simulink model "ThreeDOF_Rocket_Simulator_v4_NEW"  (R2023b)
settings: Solver=VariableStepAuto  StartTime=0.0  StopTime=30  RelTol=1e-3
libraries: shared3dof x1, simulink_extras x1, simulink x1
settings Model: Creator=giuse  LastModifiedBy=matti
settings OptimizationCC: ReuseModelBlockBuffer=off
settings DebuggingCC: UnconnectedInputMsg=warning  UnconnectedOutputMsg=warning  UnconnectedLineMsg=warning
settings ModelReferenceCC: EnableRefExpFcnMdlSchedulingChecks=on
settings RTWCC: DLArmComputeVersion=19.05

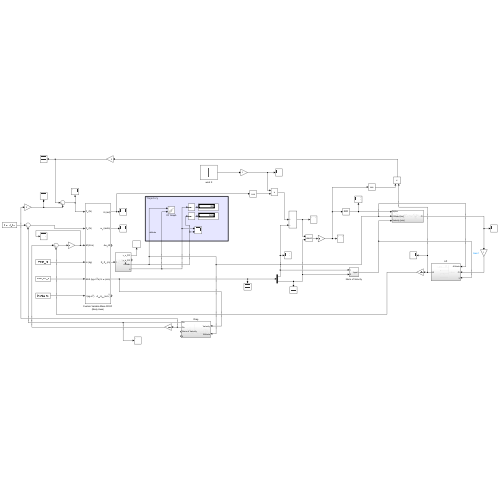
[thumbnail: Simulink's stored preview of the top-level diagram]
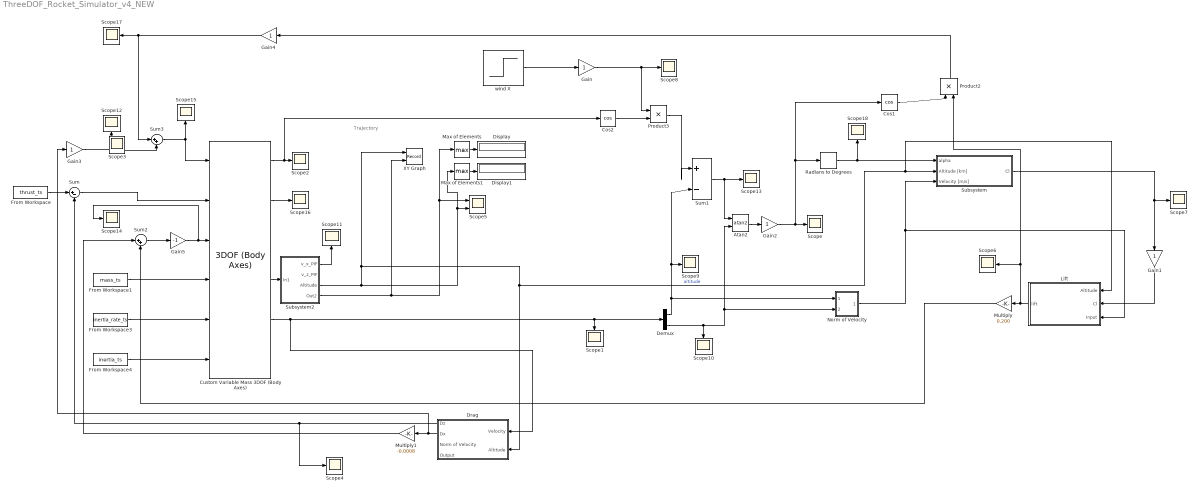
== system ThreeDOF_Rocket_Simulator_v4_NEW ==
  note: Trajectory
  Atan2 : Trigonometry  Operator=atan2
  Cos1 : Trigonometry  Operator=cos
  Cos2 : Trigonometry  Operator=cos
  Custom Variable Mass 3DOF (Body Axes) : shared3dof/3DOF (Body Axes)  units=Metric (MKS)  mtype=Custom Variable  v_ini=0  theta_ini=pi  alpha_ini=pi/2  pos_ini=[0 0]  q_ini=0  mass=1.0  mass_e=0.5  mass_f=3.0  Iyy=1.0  Iyy_e=0.5  Iyy_f=3.0  g_in=Internal  g=9.81  vre_flag=off  abi_flag=off  aMode=0  vel_statename=''  theta_statename=''  pos_statename=''  q_statename=''  mass_statename=''
  Demux : Demux  Outputs=2
  Display : Display
  Display1 : Display
  Drag : Subsystem
  From Workspace : FromWorkspace  VariableName=thrust_ts
  From Workspace1 : FromWorkspace  VariableName=mass_ts
  From Workspace3 : FromWorkspace  VariableName=inertia_rate_ts
  From Workspace4 : FromWorkspace  VariableName=inertia_ts
  Gain{,1..4} (5 alike) : Gain
  Gain5 : Gain  Gain=-1
  Lift : Subsystem
  Max of Elements : MinMax  Function=max
  Max of Elements1 : MinMax  Function=max
  Multiply : Gain  Gain=0.200
  Multiply1 : Gain  Gain=-0.0008
  Norm of Velocity : Subsystem
  Product2 : Product
  Product3 : Product
  Radians to Degrees : simulink_extras/Transformations/Radians to Degrees
  Scope{,1..4,6..18} (18 alike) : Scope
  Scope5 : Scope  NumInputPorts=2
  Subsystem : Subsystem
  Subsystem2 : Subsystem
  Sum : Sum  Inputs=|+-
  Sum1 : Sum  Inputs=|+-
  Sum2 : Sum  Inputs=|++
  Sum3 : Sum  Inputs=|++
  XY Graph : Record  FileSettingsInternal="{\"entries\":[{\"content\":{\"excelSettings\":{\"content\":{},\"type\":\"Streamout.ExcelSettings\"}},\"type\":\"Streamout.FileSettingStorage\",\"uuid\":\"\"}],\"packageUris\":[\"http:\\/\\/schema.mathworks.com\\/mf0\\/streamout_blocks\\/R2020a\"],\"version\":\"1.0\"}"  Layout=[1 1]  SignalsInternal="{\"entries\":[{\"content\":{\"signals\":[{\"content\":{\"blockPath\":[],\"dimensions\":[1],\"domain\":\"\",\"lineColor\":\"#0072bd\",\"plots\":[1],\"port\":1,\"sid\":[\"\"],\"signalID\":2529,\"signalName\":\"altitude\"},\"type\":\"RecordBlkView.Signal\",\"uuid\":\"\"},{\"content\":{\"blockPath\":[],\"dimensions\":[1],\"domain\":\"\",\"lineColor\":\"#d95319\",\"plots\":[1],\"port\":2,\"sid\":[\"\"],\"signalID\":2533,\"signalName\":\"Subsystem2:4\"},\"type\":\"RecordBlkView.Signal\",\"uuid\":\"\"}]},\"type\":\"RecordBlkView.InputSignals\",\"uuid\":\"\"}],\"packageUris\":[\"http:\\/\\/schema.mathworks.com\\/mf0\\/streamout_blocks\\/R2020a\"],\"version\":\"1.0\"}"  VisualizationBindings="{\"xyplotplugin\":{\"info\":[{\"series\":[{\"bindingParametersList\":[{\"parameter\":\"Y-Axis\",\"signalID\":2529,\"signalName\":\"altitude\"},{\"parameter\":\"X-Axis\",\"signalID\":2533,\"signalName\":\"Subsystem2:4\"}],\"seriesID\":11487}],\"subplotID\":1}]}}"  CompatibilityTag=XY
  wind X : Step  Time=0.357  After=-6  SampleTime=0
  wires:
  From Workspace1/1 -> Custom Variable Mass 3DOF (Body Axes)/4
  From Workspace4/1 -> Custom Variable Mass 3DOF (Body Axes)/6
  From Workspace/1 -> Sum/1
  Sum/1 -> Custom Variable Mass 3DOF (Body Axes)/2
  Sum2/1 -> Gain5/1
  Custom Variable Mass 3DOF (Body Axes)/4 -> Subsystem2/1(In1)
  Custom Variable Mass 3DOF (Body Axes)/5 -> Drag/1(Velocity), Demux/1, Scope1/1
  Subsystem2/3(Altitude) -> Drag/2(Altitude), Lift/1(Altitude), Subsystem/2(Altitude [km]), XY Graph/1, Max of Elements1/1, Scope5/2  "altitude"
  Subsystem2/4(Out2) -> Max of Elements/1, Scope5/1, XY Graph/2
  Max of Elements/1 -> Display/1
  Max of Elements1/1 -> Display1/1
  Drag/1(Dz) -> Scope4/1, Sum/2
  Norm of Velocity/1(Input) -> Subsystem/3(Velocity [m/s]), Lift/3(Input)
  Lift/1(lift) -> Product2/2, Scope6/1, Multiply/1
  Multiply/1 -> Sum2/2
  Custom Variable Mass 3DOF (Body Axes)/1 -> Cos2/1, Scope2/1
  wind X/1 -> Gain/1
  Gain/1 -> Product3/1, Scope8/1
  Atan2/1 -> Gain2/1
  Drag/2(Dx) -> Gain3/1, Multiply1/1
  Multiply1/1 -> Sum2/1
  Demux/2 -> Atan2/2, Norm of Velocity/2(In2), Scope10/1
  Gain1/1 -> Lift/2(Cl)
  Subsystem/1(Cl) -> Gain1/1, Scope7/1
  Subsystem2/1(v_x_PIF) -> Scope11/1
  Gain3/1 -> Sum3/2, Scope12/1
  Sum1/1 -> Scope13/1, Atan2/1
  Sum3/1 -> Custom Variable Mass 3DOF (Body Axes)/1, Scope15/1
  Cos1/1 -> Product2/1
  Product2/1 -> Gain4/1
  Gain4/1 -> Sum3/1, Scope17/1
  Cos2/1 -> Product3/2
  Demux/1 -> Norm of Velocity/1(In1), Sum1/2, Scope9/1
  Product3/1 -> Sum1/1
  Radians to Degrees/1 -> Subsystem/1(alpha), Scope18/1
  Custom Variable Mass 3DOF (Body Axes)/2 -> Scope16/1
  Gain2/1 -> Scope/1, Cos1/1, Radians to Degrees/1
  Gain5/1 -> Scope14/1, Custom Variable Mass 3DOF (Body Axes)/3
  From Workspace3/1 -> Custom Variable Mass 3DOF (Body Axes)/5

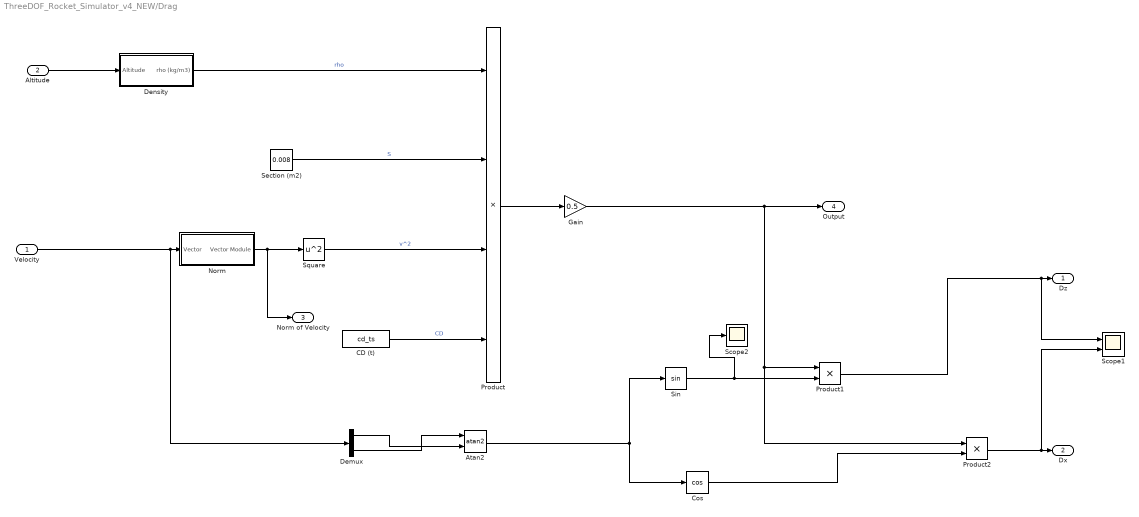
== system ThreeDOF_Rocket_Simulator_v4_NEW/Drag ==
  Velocity : Inport
  Altitude : Inport  Port=2
  Atan2 : Trigonometry  Operator=atan2
  CD (t) : FromWorkspace  VariableName=cd_ts
  Cos : Trigonometry  Operator=cos
  Demux : Demux  Outputs=2
  Density : Subsystem
  Gain : Gain  Gain=0.5
  Norm : Subsystem
  Product : Product  Inputs=4
  Product1 : Product
  Product2 : Product
  Scope1 : Scope  NumInputPorts=2
  Scope2 : Scope
  Section (m2) : Constant  Value=0.008
  Sin : Trigonometry
  Square : Math  Operator=square
  Dz : Outport
  Dx : Outport  Port=2
  Norm of Velocity : Outport  Port=3
  Output : Outport  Port=4
  wires:
  Velocity/1 -> Demux/1, Norm/1(Vector)
  Altitude/1 -> Density/1(Altitude)
  Norm/1(Vector Module) -> Norm of Velocity/1, Square/1
  Density/1(rho (kg/m3)) -> Product/1  "rho"
  Section (m2)/1 -> Product/2  "S"
  Square/1 -> Product/3  "v^2"
  Product/1 -> Gain/1
  CD (t)/1 -> Product/4  "CD"
  Sin/1 -> Scope2/1, Product1/2
  Gain/1 -> Output/1, Product2/1, Product1/1
  Cos/1 -> Product2/2
  Product2/1 -> Scope1/2, Dx/1
  Product1/1 -> Scope1/1, Dz/1
  Atan2/1 -> Sin/1, Cos/1
  Demux/2 -> Atan2/1
  Demux/1 -> Atan2/2

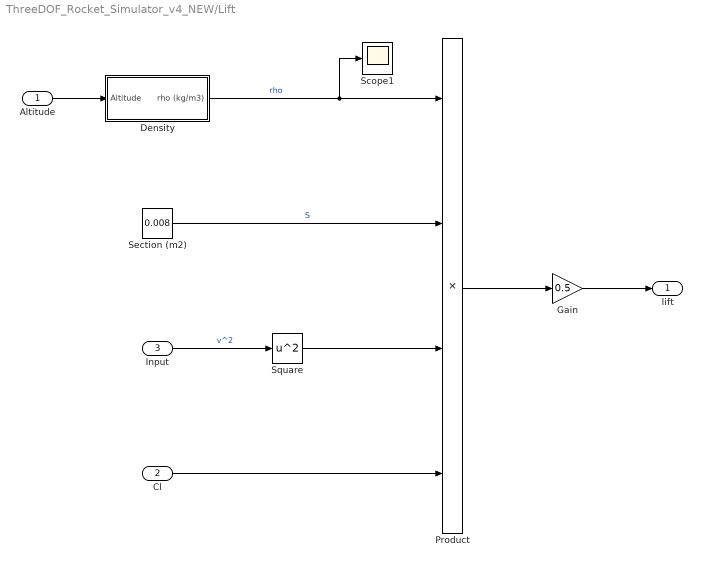
== system ThreeDOF_Rocket_Simulator_v4_NEW/Lift ==
  Altitude : Inport
  Cl : Inport  Port=2
  Input : Inport  Port=3
  Density : Subsystem
  Gain : Gain  Gain=0.5
  Product : Product  Inputs=4
  Scope1 : Scope
  Section (m2) : Constant  Value=0.008
  Square : Math  Operator=square
  lift : Outport
  wires:
  Altitude/1 -> Density/1(Altitude)
  Density/1(rho (kg/m3)) -> Scope1/1, Product/1  "rho"
  Section (m2)/1 -> Product/2  "S"
  Product/1 -> Gain/1
  Cl/1 -> Product/4
  Input/1 -> Square/1  "v^2"
  Square/1 -> Product/3
  Gain/1 -> lift/1

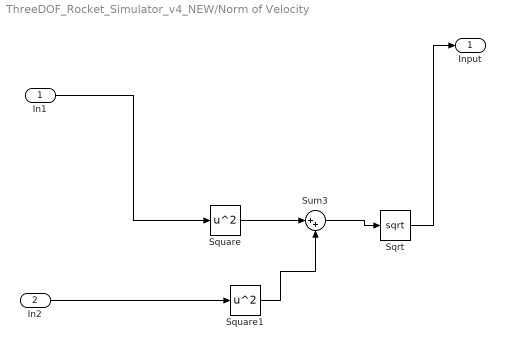
== system ThreeDOF_Rocket_Simulator_v4_NEW/Norm of Velocity ==
  In1 : Inport
  In2 : Inport  Port=2
  Sqrt : Sqrt
  Square : Math  Operator=square
  Square1 : Math  Operator=square
  Sum3 : Sum  Inputs=|++
  Input : Outport
  wires:
  Square1/1 -> Sum3/2
  Sqrt/1 -> Input/1
  Square/1 -> Sum3/1
  Sum3/1 -> Sqrt/1
  In2/1 -> Square1/1
  In1/1 -> Square/1

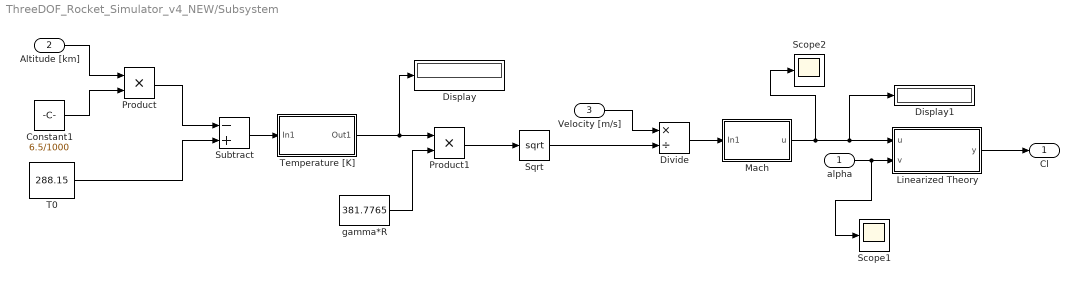
== system ThreeDOF_Rocket_Simulator_v4_NEW/Subsystem ==
  alpha : Inport
  Altitude [km] : Inport  Port=2
  Velocity [m/s] : Inport  Port=3
  Constant1 : Constant  Value=6.5/1000
  Display : Display
  Display1 : Display
  Divide : Product  Inputs=*/
  Linearized Theory : MATLAB Function  TreatAsAtomicUnit=on
  Mach : Subsystem
  Product : Product
  Product1 : Product
  Scope1 : Scope
  Scope2 : Scope
  Sqrt : Sqrt
  Subtract : Sum  Inputs=-+
  T0 : Constant  Value=288.15
  Temperature [K] : Subsystem
  gamma*R : Constant  Value=381.7765
  Cl : Outport
  wires:
  Constant1/1 -> Product/2
  Temperature [K]/1(Out1) -> Product1/1, Display/1
  T0/1 -> Subtract/2
  Subtract/1 -> Temperature [K]/1(In1)
  Mach/1(u) -> Scope2/1, Display1/1, Linearized Theory/1(u)
  Divide/1 -> Mach/1(In1)
  Sqrt/1 -> Divide/2
  Product/1 -> Subtract/1
  gamma*R/1 -> Product1/2
  Velocity [m/s]/1 -> Divide/1
  Product1/1 -> Sqrt/1
  alpha/1 -> Scope1/1, Linearized Theory/2(v)
  Linearized Theory/1(y) -> Cl/1
  Altitude [km]/1 -> Product/1

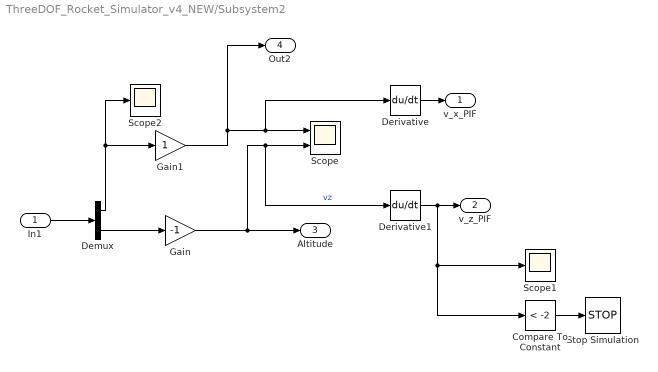
== system ThreeDOF_Rocket_Simulator_v4_NEW/Subsystem2 ==
  In1 : Inport
  Compare To Constant : simulink/Logic and Bit Operations/Compare To Constant  relop=<  const=-2  OutDataTypeStr=boolean
  Demux : Demux  Outputs=2
  Derivative : Derivative
  Derivative1 : Derivative
  Gain : Gain  Gain=-1
  Gain1 : Gain
  Scope : Scope  NumInputPorts=2
  Scope1 : Scope
  Scope2 : Scope
  Stop Simulation : Stop
  v_x_PIF : Outport
  v_z_PIF : Outport  Port=2
  Altitude : Outport  Port=3
  Out2 : Outport  Port=4
  wires:
  Demux/2 -> Gain/1
  Gain/1 -> Altitude/1, Derivative1/1, Scope/2  "vz"
  In1/1 -> Demux/1
  Demux/1 -> Scope2/1, Gain1/1
  Gain1/1 -> Out2/1, Derivative/1, Scope/1
  Derivative1/1 -> Compare To Constant/1, Scope1/1, v_z_PIF/1
  Compare To Constant/1 -> Stop Simulation/1
  Derivative/1 -> v_x_PIF/1

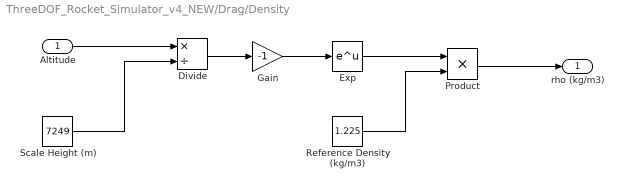
== system ThreeDOF_Rocket_Simulator_v4_NEW/Drag/Density ==
  Altitude : Inport
  Divide : Product  Inputs=*/
  Exp : Math
  Gain : Gain  Gain=-1
  Product : Product
  Reference Density (kg/m3) : Constant  Value=1.225
  Scale Height (m) : Constant  Value=7249
  rho (kg/m3) : Outport
  wires:
  Altitude/1 -> Divide/1
  Scale Height (m)/1 -> Divide/2
  Divide/1 -> Gain/1
  Gain/1 -> Exp/1
  Exp/1 -> Product/1
  Reference Density (kg/m3)/1 -> Product/2
  Product/1 -> rho (kg/m3)/1

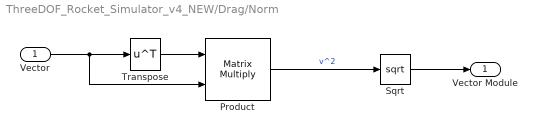
== system ThreeDOF_Rocket_Simulator_v4_NEW/Drag/Norm ==
  Vector : Inport
  Product : Product  Multiplication=Matrix(*)
  Sqrt : Sqrt
  Transpose : Math  Operator=transpose
  Vector Module : Outport
  wires:
  Vector/1 -> Product/2, Transpose/1
  Product/1 -> Sqrt/1  "v^2"
  Sqrt/1 -> Vector Module/1
  Transpose/1 -> Product/1

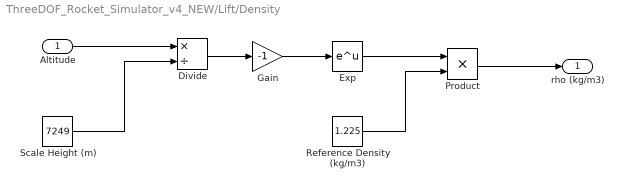
== system ThreeDOF_Rocket_Simulator_v4_NEW/Lift/Density ==
  Altitude : Inport
  Divide : Product  Inputs=*/
  Exp : Math
  Gain : Gain  Gain=-1
  Product : Product
  Reference Density (kg/m3) : Constant  Value=1.225
  Scale Height (m) : Constant  Value=7249
  rho (kg/m3) : Outport
  wires:
  Altitude/1 -> Divide/1
  Scale Height (m)/1 -> Divide/2
  Divide/1 -> Gain/1
  Gain/1 -> Exp/1
  Exp/1 -> Product/1
  Reference Density (kg/m3)/1 -> Product/2
  Product/1 -> rho (kg/m3)/1

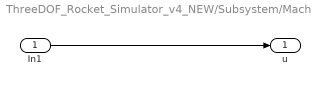
== system ThreeDOF_Rocket_Simulator_v4_NEW/Subsystem/Mach ==
  In1 : Inport
  u : Outport
  wires:
  In1/1 -> u/1

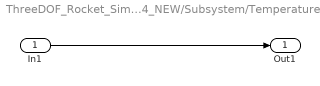
== system ThreeDOF_Rocket_Simulator_v4_NEW/Subsystem/Temperature [K] ==
  In1 : Inport
  Out1 : Outport
  wires:
  In1/1 -> Out1/1

== matlab function ThreeDOF_Rocket_Simulator_v4_NEW/Subsystem/Linearized Theory ==
  data: u input; y output; v input
function y = fcn(u,v)
%First method, linearized theory for a thin plate
if u<1
    y = ((2*pi*(v*2*pi)/360)./(sqrt(1-u.^2)))*(13500/(2*pi*(52)^2).*2);
else
    y = 4*(4*(v*pi/180))./(sqrt(u.^2-1)+2*(v*pi/180));
end
